simulink model "RIP_State_Controller"  (R2022b)
settings: Solver=VariableStepAuto  StartTime=0.0  StopTime=2  RelTol=1e-3
undefined symbols (not defined in the file): A, B, C, D, K, K_r, L, X_0
settings Model: Creator=Andrew  LastModifiedBy=Andrew

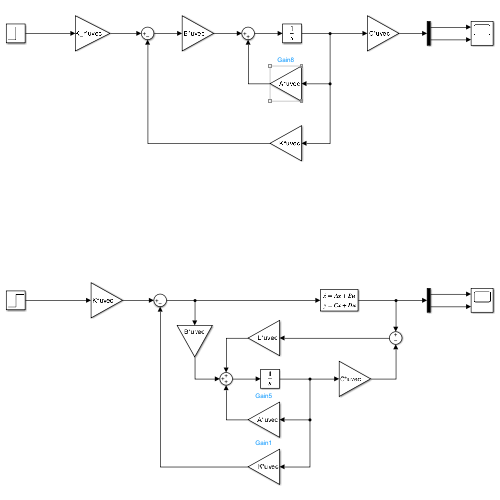
[thumbnail: Simulink's stored preview of the top-level diagram]
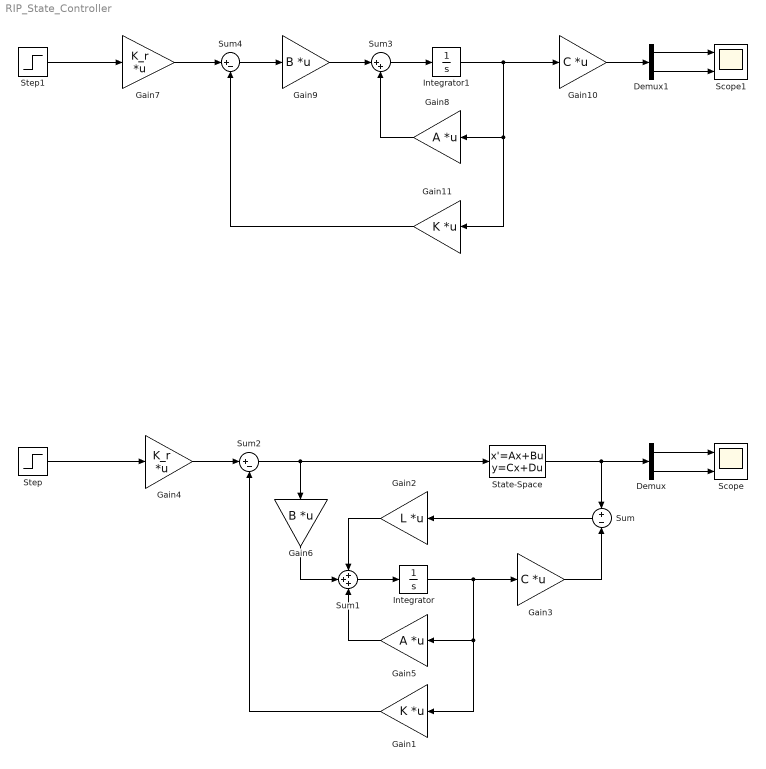
== system RIP_State_Controller ==
  Demux : Demux  Outputs=2
  Demux1 : Demux  Outputs=2
  Gain1 : Gain  Gain=K  Multiplication=Matrix(K*u) (u vector)
  Gain10 : Gain  Gain=C  Multiplication=Matrix(K*u) (u vector)
  Gain11 : Gain  Gain=K  Multiplication=Matrix(K*u) (u vector)
  Gain2 : Gain  Gain=L  Multiplication=Matrix(K*u) (u vector)
  Gain3 : Gain  Gain=C  Multiplication=Matrix(K*u) (u vector)
  Gain4 : Gain  Gain=K_r  Multiplication=Matrix(K*u) (u vector)
  Gain5 : Gain  Gain=A  Multiplication=Matrix(K*u) (u vector)
  Gain6 : Gain  Gain=B  Multiplication=Matrix(K*u) (u vector)
  Gain7 : Gain  Gain=K_r  Multiplication=Matrix(K*u) (u vector)
  Gain8 : Gain  Gain=A  Multiplication=Matrix(K*u) (u vector)
  Gain9 : Gain  Gain=B  Multiplication=Matrix(K*u) (u vector)
  Integrator : Integrator
  Integrator1 : Integrator
  Scope : Scope  NumInputPorts=2
  Scope1 : Scope  NumInputPorts=2
  State-Space : StateSpace  A=A  B=B  C=C  D=D  InitialCondition=X_0
  Step : Step  Time=0.3  SampleTime=0
  Step1 : Step  Time=0.3  SampleTime=0
  Sum : Sum  Inputs=+|-
  Sum1 : Sum  Inputs=+++
  Sum2 : Sum  Inputs=|+-
  Sum3 : Sum  Inputs=|++
  Sum4 : Sum  Inputs=|+-
  wires:
  Step/1 -> Gain4/1
  Sum/1 -> Gain2/1
  State-Space/1 -> Demux/1, Sum/1
  Gain3/1 -> Sum/2
  Sum1/1 -> Integrator/1
  Integrator/1 -> Gain3/1, Gain1/1, Gain5/1
  Gain6/1 -> Sum1/2
  Gain2/1 -> Sum1/1
  Gain5/1 -> Sum1/3
  Gain4/1 -> Sum2/1
  Sum2/1 -> Gain6/1, State-Space/1
  Gain1/1 -> Sum2/2
  Demux/1 -> Scope/1
  Demux/2 -> Scope/2
  Gain8/1 -> Sum3/2
  Step1/1 -> Gain7/1
  Sum3/1 -> Integrator1/1
  Gain9/1 -> Sum3/1
  Integrator1/1 -> Gain10/1, Gain11/1, Gain8/1
  Demux1/2 -> Scope1/2
  Demux1/1 -> Scope1/1
  Gain10/1 -> Demux1/1
  Gain7/1 -> Sum4/1
  Sum4/1 -> Gain9/1
  Gain11/1 -> Sum4/2
